simulink model "r2b2xpfb14mcr17b"  (R2012b)
settings: Solver=VariableStepDiscrete  SolverMode=SingleTasking  StartTime=0.0  StopTime=10.0  RelTol=1e-3
undefined symbols (not defined in the file): bit_reverse, pfb_coeff_gen_calc
libraries: xbsIndex_r4 x7914, casper_library_misc x51, casper_library_delays x18, xps_library x4
(part 89 of 104)

== system r2b2xpfb14mcr17b/fft_biplex_2by2_real/fft_biplex_real_2x2/biplex_core/fft_stage_13/butterfly_direct/twiddle/coeff_gen/cosin ==
  theta : Inport
  misci : Inport  Port=2
  Constant4 : xbsIndex_r4/Constant  const=0  gui_display_data_type=Fixed-point  arith_type=Unsigned  n_bits=1  bin_pt=0  preci_type=Single  exp_width=8  frac_width=24  explicit_period=on  period=1  equ=P=C  opselect=C  inp2=PCIN>>17  opr=+  inp1=P  carry=CIN  dbl_ovrd=off  block_type=constant
  Constant5 : xbsIndex_r4/Constant  const=0  gui_display_data_type=Fixed-point  arith_type=Unsigned  n_bits=1  bin_pt=0  preci_type=Single  exp_width=8  frac_width=24  explicit_period=on  period=1  equ=P=C  opselect=C  inp2=PCIN>>17  opr=+  inp1=P  carry=CIN  dbl_ovrd=off  block_type=constant
  Delay : xbsIndex_r4/Delay  rst=off  infoeditControl=Selection of Reset will increase slice count due to use of real FFs and instead of SRLs  en=off  latency=bram_latency  dbl_ovrd=off  reg_retiming=on  block_type=delay
  Delay10 : xbsIndex_r4/Delay  rst=off  infoeditControl=Selection of Reset will increase slice count due to use of real FFs and instead of SRLs  en=off  latency=bram_latency  dbl_ovrd=off  reg_retiming=on  block_type=delay
  Delay8 : xbsIndex_r4/Delay  rst=off  infoeditControl=Selection of Reset will increase slice count due to use of real FFs and instead of SRLs  en=off  latency=bram_latency  dbl_ovrd=off  reg_retiming=on  block_type=delay
  ROM : xbsIndex_r4/ROM  depth=2^(12)  initVector=[34359476224 34359738267 34359738167 34359738066 34359737966 34359737865 34359737765 34359475520 34359475420 34359213175 34358950931 34358688686 34358426442 34358164197 34357901953 34357639708 34357377464 34357115219 34356852975 34356328586 34356066341 34355541953 34355017564 34354755320 34354230931 34353706543 34353182154 34352657766 34352133377 34351608989 34350822456 34350298068 34349773679 34348987147 34348200614 34347676226 34346889693 34346103161 34345316628 34344530096 34343743563 34342957031 34342170498 34341383966 34340335289 34339548757 34338500081 34337713548 34336664872 34335616195 34334829663 34333780986 34332732310 34331683633 34330634957 34329324136 34328275460 34327226784 34325915963 34324867287 34323556466 34322507790 34321196969 34319886149 34318575329 34317264508 34315953688 34314642867 34313332047 34311759083 34310448262 34309137442 34307564477 34306253657 34304680693 34303107728 34301534764 34299961800 34298650979 34296815871 34295242907 34293669942 34292096978 34290261870 34288688905 34287115941 34285280833 34283445724 34281872760 34280037652 34278202543 34276367435 34274532327 34272697219 34270599966 34268764858 34266929750 34264832497 34262997389 34260900137 34259065029 34256967777 34254870524 34252773272 34250676020 34248578768 34246481515 34244384263 34242287011 34239927615 34237830363 34235470967 34233373714 34231014318 34228654922 34226295526 34224198274 34221838878 34219479482 34216857941 34214498545 34212139149 34209779753 34207158213 34204798817 34202177277 34199555737 34197196341 34194574801 34191953261 34189331721 34186710181 34184088641 34181467101 34178583417 34175961877 34173340337 34170456653 34167572969 34164951429 34162067745 34159184061 34156300377 34153416693 34150533009 34147649325 34144765641 34141881957 34138736129 34135852445 34132968762 34129822934 34126677106 34123793422 34120647594 34117501766 34114355939 34111210111 34108064283 34104918455 34101510483 34098364656 34095218828 34091810856 34088402884 34085257057 34081849085 34078441113 34075033141 34071625170 34068217198 34064809226 34061401255 34057993283 34054323167 34050915196 34047507224 34043837109 34040166993 34036759021 34033088906 34029418790 34025748675 34022078559 34018408444 34014738328 34010806069 34007135953 34003465838 33999533578 33995863463 33991931203 33987998944 33984328828 33980396569 33976464309 33972532050 33968599791 33964405387 33960473128 33956540869 33952346465 33948414206 33944219803 33940287543 33936093140 33931898737 33927966477 33923772074 33919577671 33915121124 33910926720 33906732317 33902537914 33898081367 33893886964 33889430417 33885236013 33880779466 33876322919 33871866372 33867671969 33863215422 33858496731 33854040184 33849583637 33845127090 33840408399 33835951852 33831233161 33826776614 33822057923 33817339232 33812882685 33808163994 33803445303 33798726612 33793745777 33789027086 33784308395 33779589705 33774608870 33769890179 33764909344 33759928509 33755209819 33750228984 33745248149 33740267314 33735286480 33730305645 33725324810 33720081832 33715100997 33710120162 33704877184 33699634205 33694653371 33689410392 33684167413 33678924435 33673681456 33668438478 33663195499 33657952521 33652709542 33647466564 33641961441 33636718463 33631213341 33625970362 33620465240 33614960117 33609454995 33603949873 33598444751 33592939628 33587434506 33581929384 33576162117 33570656995 33565151873 33559384607 33553617341 33548112218 33542344952 33536577686 33530810420 33525043154 33519275888 33513508622 33507741356 33501974090 33495944680 33490177414 33484148004 33478380738 33472351328 33466321918 33460292508 33454263098 33448495832 33442204278 33436174869 33430145459 33424116049 33418086639 33411795085 33405765676 33399474122 33393182568 33387153159 33380861605 33374570051 33368278498 33361986944 33355695390 33349403837 33343112283 33336558586 33330267032 33323713335 33317421781 33310868084 33304576530 33298022833 33291469135 33284915438 33278361741 33271808043 33265254346 33258700649 33251884807 ...(+44726 chars)]  distributed_mem=Block RAM  rst=off  init_reg=0  en=off  latency=bram_latency  gui_display_data_type=Fixed-point  arith_type=Unsigned  n_bits=n_bits*2  bin_pt=0  preci_type=Single  exp_width=8  frac_width=24  dbl_ovrd=off  optimize=Speed  use_rpm=on  block_type=sprom
  Terminator : Terminator
  Terminator1 : Terminator
  Terminator4 : Terminator
  add_convert0 : Subsystem
  add_convert1 : Subsystem
  assert : xbsIndex_r4/Assert  assert_type=on  type_source=Explicitly  gui_display_data_type=Fixed-point  arith_type=Unsigned  n_bits=12  bin_pt=0  preci_type=Single  exp_width=8  frac_width=24  assert_rate=off  rate_source=Explicitly  period=1  output_port=on  block_type=assert
  c_to_ri : casper_library_misc/c_to_ri  n_bits=n_bits  bin_pt=bin_pt
  invert0 : Subsystem  mask{n_bits=n_bits, bin_pt=bin_pt, neg_latency=neg_latency, mux_latency=mux_latency}
      mask prompts: n_bits "bit width"; bin_pt "binary point"; neg_latency "negate latency"; mux_latency "mux latency"
  invert1 : Subsystem  mask{n_bits=n_bits, bin_pt=bin_pt, neg_latency=neg_latency, mux_latency=mux_latency}
      mask prompts: n_bits "bit width"; bin_pt "binary point"; neg_latency "negate latency"; mux_latency "mux latency"
  cos : Outport
  -sin : Outport  Port=2
  misco : Outport  Port=3
  wires:
  theta/1 -> assert/1
  assert/1 -> add_convert0/1(theta), add_convert1/1(theta)
  Constant4/1 -> add_convert0/2(misci)
  add_convert0/3(misco) -> Terminator/1
  misci/1 -> add_convert1/2(misci)
  add_convert1/3(misco) -> Delay/1
  add_convert0/2(add) -> ROM/1
  add_convert1/2(add) -> Terminator4/1
  ROM/1 -> c_to_ri/1
  add_convert1/1(negate) -> Delay8/1
  add_convert0/1(negate) -> Delay10/1
  Delay10/1 -> invert0/1(negate)
  Constant5/1 -> invert0/3(misci)
  c_to_ri/1 -> invert0/2(in)
  Delay8/1 -> invert1/1(negate)
  c_to_ri/2 -> invert1/2(in)
  invert0/2(misco) -> Terminator1/1
  Delay/1 -> invert1/3(misci)
  invert0/1(out) -> cos/1
  invert1/2(misco) -> misco/1
  invert1/1(out) -> -sin/1
